simulink model "Tactor_NoTask _bkp"  (R2022b)
settings: Solver=FixedStepDiscrete  StartTime=0.0  StopTime=Inf  FixedStep=0.001  RelTol=1e-3  EnableMultiTasking=on
PreLoadFcn:
  | parambus = Simulink.Bus;
  | idx = 0;
  | 
  | idx = idx + 1;
  | parambus.Elements(idx) = Simulink.BusElement;
  | parambus.Elements(idx).Name = 'StimOn';
  | parambus.Elements(idx).DataType = 'uint8';
  | parambus.Elements(idx).Dimensions = [1, 1];
  | 
  | idx = idx + 1;
  | parambus.Elements(idx) = Simulink.BusElement;
  | parambus.Elements(idx).Name = 'DelayPeriod';
  | parambus.Elements(idx).DataType = 'uint16';
  | parambus.Elements(idx).Dimensions = [1, 2];
  | 
  | idx = idx + 1;
  | parambus.Elements(idx) = Simulink.BusElement;
  | parambus.Elements(idx).Name = 'StimDuration';
  | parambus.Elements(idx).DataType = 'uint16';
  | parambus.Elements(idx).Dimensions = [1, 1];
  | 
  | %%
  | 
  | FileLoggerEntry = Simulink.Bus;
  | FileLoggerEntry.Elements(1) = Simulink.BusElement;
  | FileLoggerEntry.Elements(1).Name = 'FileType';
  | FileLoggerEntry.Elements(1).DataType = 'uint8';
  | FileLoggerEntry.Elements(1).Dimensions = [1, 1];
  | FileLoggerEntry.Elements(2) = Simulink.BusElement;
  | FileLoggerEntry.Elements(2).Name = 'FieldName';
  | FileLoggerEntry.Elements(2).DataType = 'uint8';
  | FileLoggerEntry.Elements(2).Dimensions = [1, 20];
  | FileLoggerEntry.Elements(3) = Simulink.BusElement;
  | FileLoggerEntry.Elements(3).Name = 'DataType';
  | FileLoggerEntry.Elements(3).DataType = 'uint8';
  | FileLoggerEntry.Elements(3).Dimensions = [1, 6];
  | FileLoggerEntry.Elements(4) = Simulink.BusElement;
  | FileLoggerEntry.Elements(4).Name = 'NumElements';
  | FileLoggerEntry.Elements(4).DataType = 'uint8';
  | FileLoggerEntry.Elements(4).Dimensions = [1, 1];
  | FileLoggerEntry.Elements(5) = Simulink.BusElement;
  | FileLoggerEntry.Elements(5).Name = 'Data';
  | FileLoggerEntry.Elements(5).DataType = 'double';
  | FileLoggerEntry.Elements(5).Dimensions = [1, 255];
undefined symbols (not defined in the file): Ended, Single
libraries: slrealtimeiplib x6, speedgoatlib_IO191 x3, slrealtimeseriallib x2
settings Model: Creator=irwin  LastModifiedBy=l-zirwin
settings SolverCC: ConcurrentTasks=on  AlgebraicLoopSolver=TrustRegion  PositivePriorityOrder=on  InsertRTBMode=Never (minimum delay)
settings DataIOCC: SaveFormat=Array  SaveState=on  SignalLoggingName=logsOut
settings OptimizationCC: BlockReduction=off  BooleanDataType=off  OptimizeBlockIOStorage=off  BufferReuse=off  GlobalBufferReuse=off  ExpressionFolding=off  LocalBlockOutputs=off  InitFltsAndDblsToZero=on  OptimizeDataStoreBuffers=off  BusAssignmentInplaceUpdate=off
settings DebuggingCC: SaveWithParameterizedLinksMsg=none  UnderspecifiedInitializationDetection=Classic  MergeDetectMultiDrivingBlocksExec=none  CheckExecutionContextPreStartOutputMsg=on  SignalResolutionControl=TryResolveAllWithWarning  TasksWithSamePriorityMsg=none  UnconnectedInputMsg=warning  UnconnectedOutputMsg=warning  UnconnectedLineMsg=warning  SFUnexpectedBacktrackingDiag=warning  SFNoUnconditionalDefaultTransitionDiag=warning  SFExecutionAtInitializationDiag=none  SFMachineParentedDataDiag=warning  ArithmeticOperatorsInVariantConditions=warning
settings HardwareCC: ProdBitPerLong=64  ProdLongLongMode=on  ProdHWDeviceType=Intel->x86-64 (Linux 64)
settings ModelReferenceCC: EnableRefExpFcnMdlSchedulingChecks=on  PropagateSignalLabelsOutOfModel=off
settings SFSimCC: SimUseLocalCustomCode=off  SimTargetLang=C++
settings RTWCC: Description=Simulink Real-Time  SystemTargetFile=slrealtime.tlc  TemplateMakefile=slrealtime_default_tmf  RTWUseLocalCustomCode=off  Toolchain=Simulink Real-Time Toolchain  BuildConfiguration=Faster Runs  CodeExecutionProfiling=on  TargetLang=C++  DLArmComputeVersion=19.05
settings CodeAppCC: StateflowObjectComments=on
settings SimulinkRealTimeTargetCC: MATLABClassNameForMDSCustomization=Simulink.SoftwareTarget.GRTCustomization  UseGCCFastMath=on
settings ConfigComp: CovMetricSettings=dw  CovSaveCumulativeToWorkspaceVar=on  CovSaveSingleToWorkspaceVar=on  CovExternalEMLEnable=off  CovSFcnEnable=off

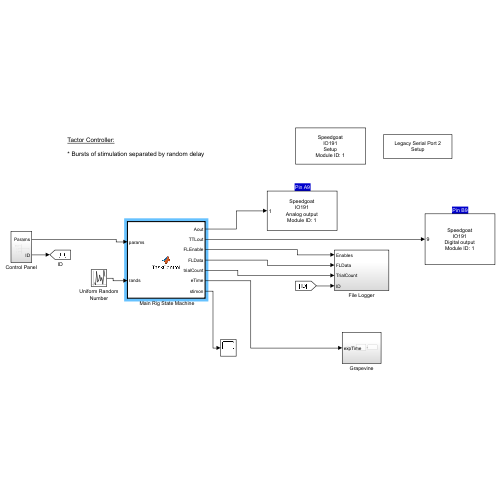
[thumbnail: Simulink's stored preview of the top-level diagram]
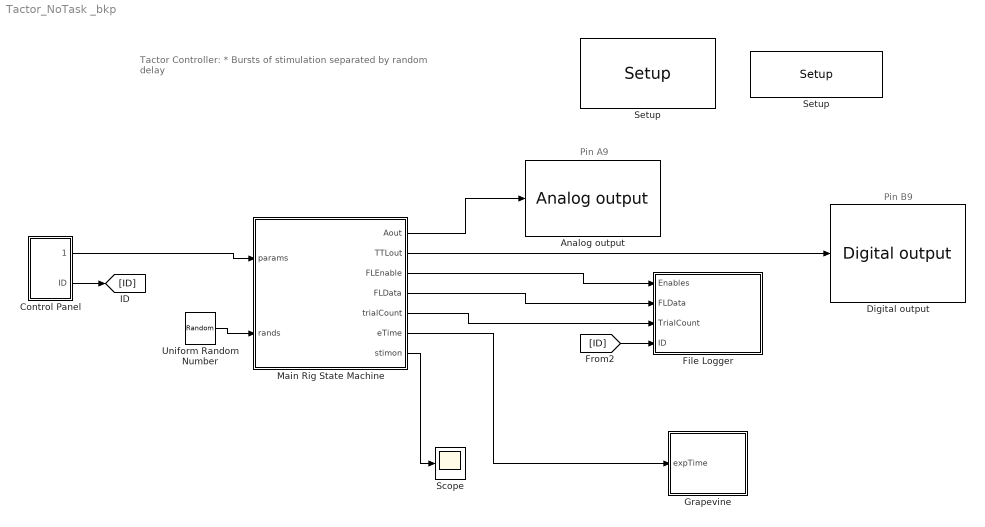
== system Tactor_NoTask _bkp ==
  note: Pin A9
  note: Pin B9
  note: Tactor Controller:
      |
      | * Bursts of stimulation separated by random delay
  " Main Rig State Machine" : MATLAB Function  TreatAsAtomicUnit=on
  "Analog output " : speedgoatlib_IO191/Analog output   parModuleId=1  parSampleTime=-1  parPciSlot=-1  parDacChannels=1  parModuleType=1  parDacRanges=5  parDacInitValues=0  parDacResets=1
      settings: SourceProductName=Simulink Real-Time: Speedgoat I/O Blockset
  Control Panel : Subsystem
  "Digital output " : speedgoatlib_IO191/Digital output   parModuleId=1  parSampleTime=-1  parPciSlot=-1  parDoChannels=9  parDoInitValues=0  parDoResets=1
      settings: SourceProductName=Simulink Real-Time: Speedgoat I/O Blockset
  File Logger : Subsystem
  Grapevine : Subsystem
  Scope : Scope
  Setup : slrealtimeseriallib/Mainboard/Setup  port=Legacy Serial Port 2  baud=115200  width=8  nstop=1  parity=None  ctsmode=off
  "Setup " : speedgoatlib_IO191/Setup   parModuleId=1  parPciSlot=-1  parTriggerSignal=TTL  parAdcChannels=1  parAdcRanges=3  parAdcChannel1=on  parAdcChannel2=off  parAdcChannel3=off  parAdcChannel4=off  parAdcChannel5=off  parAdcChannel6=off  parAdcChannel7=off  parAdcChannel8=off  parAdcMode=Single-Ended  parAdcRate=100000  parAdcRange11=+-10.24 V  parAdcRange21=+-24.576 V  parAdcRange12=+-10.24 V  parAdcRange22=+-24.576 V  parAdcRange13=+-10.24 V  parAdcRange23=+-24.576 V  parAdcRange14=+-10.24 V  parAdcRange24=+-24.576 V  parAdcRange15=+-10.24 V  parAdcRange25=+-24.576 V  parAdcRange16=+-10.24 V  parAdcRange26=+-24.576 V  parAdcRange17=+-10.24 V  parAdcRange27=+-24.576 V  parAdcRange18=+-10.24 V  parAdcRange28=+-24.576 V  parDacChannels=1  parDacChannel1=on  parDacChannel2=off  parDacChannel3=off  parDacChannel4=off  parDacMode=Single-Ended  parDacRanges=5  parDacInitValues=0  parDacResets=1  parDacRange1=+-2.5 V  parDacInitValue1=0  parDacReset1=on  parDacRange2=+-10 V  parDacInitValue2=0  parDacReset2=on  parDacRange3=+-10 V  parDacInitValue3=0  parDacReset3=on  parDacRange4=+-10 V  parDacInitValue4=0  parDacReset4=on  parDiChannels=[1 2 3 4 5 6 7 8 10 11 12 13 14 15 16]  parDoChannels=9  parDioFirstControl=2  parDioSecondControl=0  parDioChannel1=In  parExtra1=I  parExtra2=I  parExtra3=I  parDioChannel2=Out  parDioChannel3=In  parDioChannel4=In  parDioChannel5=In  parDioChannel6=In  parDioChannel7=In  parDioChannel8=In  parDioChannel9=In  parDoInitValues=[0 0 0 0]  parDoResets=[1 1 1 1]  parDoInitValue1=0  parDoReset1=on  parDoInitValue2=0  parDoReset2=on  parDoInitValue3=0  parDoReset3=on  parDoInitValue4=0  parDoReset4=on  parDoInitValue5=0  parDoReset5=on  parDoInitValue6=0  parDoReset6=on  parDoInitValue7=0  parDoReset7=on  parDoInitValue8=0  parDoReset8=on  parDoInitValue9=0  parDoReset9=on  parDoInitValue10=0  parDoReset10=on  parDoInitValue11=0  parDoReset11=on  parDoInitValue12=0  parDoReset12=on  parDoInitValue13=0  parDoReset13=on  parDoInitValue14=0  parDoReset14=on  parDoInitValue15=0  parDoReset15=on  parDoInitValue16=0  parDoReset16=on
      settings: SourceProductName=Simulink Real-Time: Speedgoat I/O Blockset
  Uniform Random Number : UniformRandomNumber  Minimum=[0]  Maximum=[1]  SampleTime=.001
  wires:
  " Main Rig State Machine"/3(FLEnable) -> File Logger/1(Enables)
  " Main Rig State Machine"/4(FLData) -> File Logger/2(FLData)
  " Main Rig State Machine"/5(trialCount) -> File Logger/3(TrialCount)
  Control Panel/2(ID) -> [ID]
  [ID] -> File Logger/4(ID)
  Control Panel/1(Params) -> " Main Rig State Machine"/1(params)
  Uniform Random Number/1 -> " Main Rig State Machine"/2(rands)
  " Main Rig State Machine"/1(Aout) -> "Analog output "/1
  " Main Rig State Machine"/2(TTLout) -> "Digital output "/1
  " Main Rig State Machine"/6(eTime) -> Grapevine/1(expTime)
  " Main Rig State Machine"/7(stimon) -> Scope/1

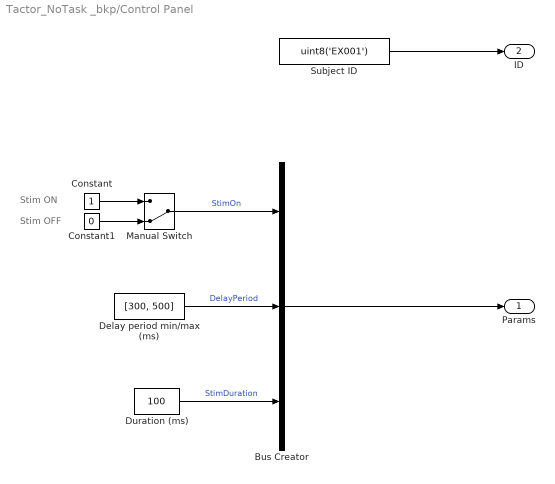
== system Tactor_NoTask _bkp/Control Panel ==
  note: Stim ON
  note: Stim OFF
  Bus Creator : BusCreator  Inputs=3  OutDataTypeStr=Bus: parambus  NonVirtualBus=on
  Constant : Constant  OutDataTypeStr=uint8
  Constant1 : Constant  Value=0  OutDataTypeStr=uint8
  Delay period min/max (ms) : Constant  Value=[300, 500]  OutDataTypeStr=uint16
  Duration (ms) : Constant  Value=100  OutDataTypeStr=uint16
  Manual Switch : ManualSwitch  CurrentSetting=0
  Subject ID : Constant  Value=uint8('EX001')  OutDataTypeStr=uint8
  Params : Outport
  ID : Outport  Port=2
  wires:
  Delay period min/max (ms)/1 -> Bus Creator/2  "DelayPeriod"
  Manual Switch/1 -> Bus Creator/1  "StimOn"
  Constant1/1 -> Manual Switch/2
  Constant/1 -> Manual Switch/1
  Bus Creator/1 -> Params/1
  Duration (ms)/1 -> Bus Creator/3  "StimDuration"
  Subject ID/1 -> ID/1

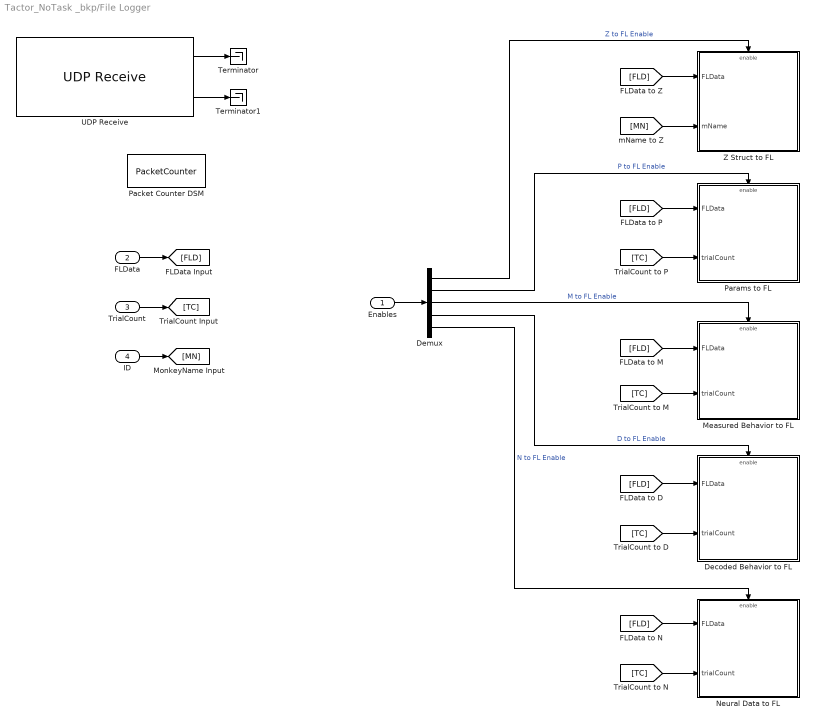
== system Tactor_NoTask _bkp/File Logger ==
  Enables : Inport  OutDataTypeStr=uint8  PortDimensions=[1 5]
  FLData : Inport  Port=2  OutDataTypeStr=Bus: FileLoggerEntry
  TrialCount : Inport  Port=3
  ID : Inport  Port=4
  Decoded Behavior to FL : Subsystem
  Demux : Demux  Outputs=5
  Measured Behavior to FL : Subsystem
  Neural Data to FL : Subsystem
  Packet Counter DSM : DataStoreMemory  DataStoreName=PacketCounter  WriteAfterWriteMsg=warning  ShowAdditionalParam=off  OutDataTypeStr=uint32  Dimensions=1
  Params to FL : Subsystem
  Terminator : Terminator
  Terminator1 : Terminator
  UDP Receive : slrealtimeiplib/UDP Receive  useHostTargetConn=off  ipAddress='192.168.8.1'  localPort=11114  rcvWidth=16  rcvFmAny=off  fmAddress='192.168.8.7'  sampleTime=-1  enableMessage=off  maxPackets=1
  Z Struct to FL : Subsystem
  wires:
  TrialCount/1 -> [TC]
  FLData/1 -> [FLD]
  [FLD] -> Z Struct to FL/1(FLData)
  [FLD] -> Params to FL/1(FLData)
  [FLD] -> Measured Behavior to FL/1(FLData)
  [FLD] -> Decoded Behavior to FL/1(FLData)
  [FLD] -> Neural Data to FL/1(FLData)
  [TC] -> Params to FL/2(trialCount)
  [TC] -> Measured Behavior to FL/2(trialCount)
  [TC] -> Decoded Behavior to FL/2(trialCount)
  [TC] -> Neural Data to FL/2(trialCount)
  Enables/1 -> Demux/1
  Demux/3 -> Measured Behavior to FL/Enable  "M to FL Enable"
  Demux/4 -> Decoded Behavior to FL/Enable  "D to FL Enable"
  Demux/5 -> Neural Data to FL/Enable  "N to FL Enable"
  Demux/2 -> Params to FL/Enable  "P to FL Enable"
  Demux/1 -> Z Struct to FL/Enable  "Z to FL Enable"
  ID/1 -> [MN]
  [MN] -> Z Struct to FL/2(mName)
  UDP Receive/2 -> Terminator1/1
  UDP Receive/1 -> Terminator/1

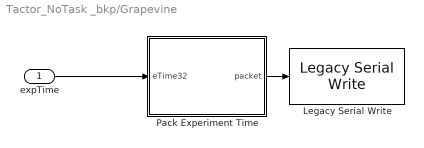
== system Tactor_NoTask _bkp/Grapevine ==
  expTime : Inport
  Legacy Serial Write : slrealtimeseriallib/Mainboard/Legacy Serial Write  port=Legacy Serial Port 2  dtype=count+32 bit uint  sampletime=-1
  Pack Experiment Time : MATLAB Function  TreatAsAtomicUnit=on
  wires:
  expTime/1 -> Pack Experiment Time/1(eTime32)
  Pack Experiment Time/1(packet) -> Legacy Serial Write/1

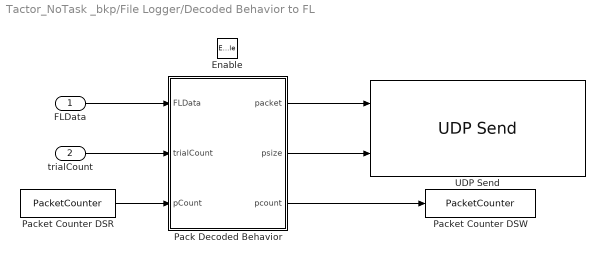
== system Tactor_NoTask _bkp/File Logger/Decoded Behavior to FL ==
  FLData : Inport
  trialCount : Inport  Port=2
  Enable : EnablePort
  Pack Decoded Behavior : MATLAB Function  TreatAsAtomicUnit=on
  Packet Counter DSR : DataStoreRead  DataStoreName=PacketCounter  SampleTime=.001  IndexOptions=Index vector (dialog)  Indices=1  OutputSizes=1
  Packet Counter DSW : DataStoreWrite  DataStoreName=PacketCounter  IndexOptions=Index vector (dialog)  Indices=1  OutputSizes=1
  UDP Send : slrealtimeiplib/UDP Send  useHostTargetConn=off  toAddress='192.168.8.7'  toPort=11114  sampleTime=-1  enableMessage=off  ipAddress='192.168.8.1'  localPort=11114
  wires:
  FLData/1 -> Pack Decoded Behavior/1(FLData)
  trialCount/1 -> Pack Decoded Behavior/2(trialCount)
  Packet Counter DSR/1 -> Pack Decoded Behavior/3(pCount)
  Pack Decoded Behavior/1(packet) -> UDP Send/1
  Pack Decoded Behavior/3(pcount) -> Packet Counter DSW/1
  Pack Decoded Behavior/2(psize) -> UDP Send/2

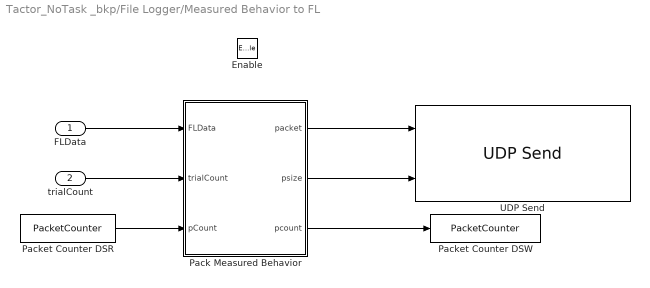
== system Tactor_NoTask _bkp/File Logger/Measured Behavior to FL ==
  FLData : Inport
  trialCount : Inport  Port=2
  Enable : EnablePort
  Pack Measured Behavior : MATLAB Function  TreatAsAtomicUnit=on
  Packet Counter DSR : DataStoreRead  DataStoreName=PacketCounter  SampleTime=.001  IndexOptions=Index vector (dialog)  Indices=1  OutputSizes=1
  Packet Counter DSW : DataStoreWrite  DataStoreName=PacketCounter  IndexOptions=Index vector (dialog)  Indices=1  OutputSizes=1
  UDP Send : slrealtimeiplib/UDP Send  useHostTargetConn=off  toAddress='192.168.8.7'  toPort=11114  sampleTime=-1  enableMessage=off  ipAddress='192.168.8.1'  localPort=11114
  wires:
  FLData/1 -> Pack Measured Behavior/1(FLData)
  trialCount/1 -> Pack Measured Behavior/2(trialCount)
  Packet Counter DSR/1 -> Pack Measured Behavior/3(pCount)
  Pack Measured Behavior/3(pcount) -> Packet Counter DSW/1
  Pack Measured Behavior/1(packet) -> UDP Send/1
  Pack Measured Behavior/2(psize) -> UDP Send/2

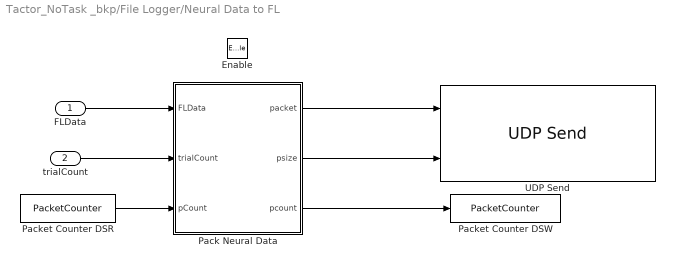
== system Tactor_NoTask _bkp/File Logger/Neural Data to FL ==
  FLData : Inport
  trialCount : Inport  Port=2
  Enable : EnablePort
  Pack Neural Data : MATLAB Function  TreatAsAtomicUnit=on
  Packet Counter DSR : DataStoreRead  DataStoreName=PacketCounter  SampleTime=.001  IndexOptions=Index vector (dialog)  Indices=1  OutputSizes=1
  Packet Counter DSW : DataStoreWrite  DataStoreName=PacketCounter  IndexOptions=Index vector (dialog)  Indices=1  OutputSizes=1
  UDP Send : slrealtimeiplib/UDP Send  useHostTargetConn=off  toAddress='192.168.8.7'  toPort=11114  sampleTime=-1  enableMessage=off  ipAddress='192.168.8.1'  localPort=11114
  wires:
  FLData/1 -> Pack Neural Data/1(FLData)
  trialCount/1 -> Pack Neural Data/2(trialCount)
  Packet Counter DSR/1 -> Pack Neural Data/3(pCount)
  Pack Neural Data/3(pcount) -> Packet Counter DSW/1
  Pack Neural Data/1(packet) -> UDP Send/1
  Pack Neural Data/2(psize) -> UDP Send/2

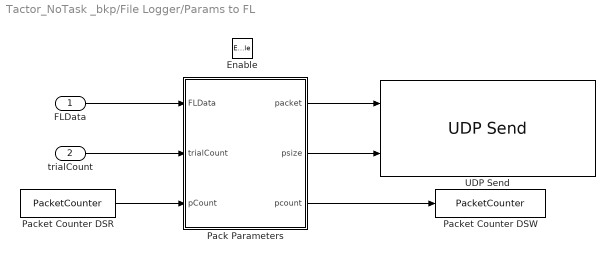
== system Tactor_NoTask _bkp/File Logger/Params to FL ==
  FLData : Inport
  trialCount : Inport  Port=2
  Enable : EnablePort
  Pack Parameters : MATLAB Function  TreatAsAtomicUnit=on
  Packet Counter DSR : DataStoreRead  DataStoreName=PacketCounter  SampleTime=.001  IndexOptions=Index vector (dialog)  Indices=1  OutputSizes=1
  Packet Counter DSW : DataStoreWrite  DataStoreName=PacketCounter  IndexOptions=Index vector (dialog)  Indices=1  OutputSizes=1
  UDP Send : slrealtimeiplib/UDP Send  useHostTargetConn=off  toAddress='192.168.8.7'  toPort=11114  sampleTime=-1  enableMessage=off  ipAddress='192.168.8.1'  localPort=11114
  wires:
  FLData/1 -> Pack Parameters/1(FLData)
  trialCount/1 -> Pack Parameters/2(trialCount)
  Packet Counter DSR/1 -> Pack Parameters/3(pCount)
  Pack Parameters/1(packet) -> UDP Send/1
  Pack Parameters/2(psize) -> UDP Send/2
  Pack Parameters/3(pcount) -> Packet Counter DSW/1

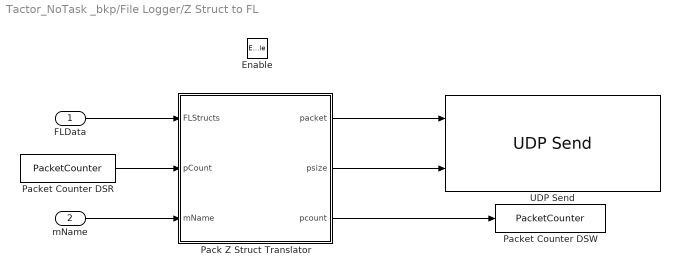
== system Tactor_NoTask _bkp/File Logger/Z Struct to FL ==
  FLData : Inport
  mName : Inport  Port=2
  Enable : EnablePort
  Pack Z Struct Translator : MATLAB Function  TreatAsAtomicUnit=on
  Packet Counter DSR : DataStoreRead  DataStoreName=PacketCounter  SampleTime=.001  IndexOptions=Index vector (dialog)  Indices=1  OutputSizes=1
  Packet Counter DSW : DataStoreWrite  DataStoreName=PacketCounter  IndexOptions=Index vector (dialog)  Indices=1  OutputSizes=1
  UDP Send : slrealtimeiplib/UDP Send  useHostTargetConn=off  toAddress='192.168.8.7'  toPort=11114  sampleTime=-1  enableMessage=off  ipAddress='192.168.8.1'  localPort=11114
  wires:
  FLData/1 -> Pack Z Struct Translator/1(FLStructs)
  Packet Counter DSR/1 -> Pack Z Struct Translator/2(pCount)
  mName/1 -> Pack Z Struct Translator/3(mName)
  Pack Z Struct Translator/3(pcount) -> Packet Counter DSW/1
  Pack Z Struct Translator/1(packet) -> UDP Send/1
  Pack Z Struct Translator/2(psize) -> UDP Send/2

== matlab function Tactor_NoTask _bkp/Grapevine/Pack Experiment Time ==
  data: eTime32 input uint32 size=1; packet output uint32 size=[1,5]
function packet = TypecastETime(eTime32)


packet = uint32([4, typecast(eTime32, 'uint8')]);

== matlab function Tactor_NoTask _bkp/ Main Rig State Machine ==
  data: Aout output double size=1; TTLout output double size=1; params input; rands input; FLEnable output; FLData output Bus: FileLoggerEntry; trialCount output; eTime output uint32 size=1; stimon output
function [Aout, TTLout, FLEnable, FLData, trialCount, eTime, stimon] = TaskControl(params, rands)

persistent exp_state trial_state exp_time trial_time trial_count intparams extparams...
           FLStruct

if (isempty(exp_state))
    exp_state = uint8(0);           % Experiment state variable
    trial_state = uint8(0);         % Trial state variable
    exp_time = uint32(0);           % Current experiment time
    trial_time = uint32(0);         % Current trial time
    trial_count = uint16(0);        % Count of the trials in the current run
    extparams = params;             % Initialize parameters to incoming struct
    FLStruct = genFLStruct();       % Struct array for File Logger data

    intparams = struct('DelayTime', uint16(0), ...          % delay period (ms)
                       'BlankTrial', uint8(0));          % indicator that stim was turned off

end

%%%%%%%%%%%%%%%%%%%%%%%%%%%%%%% Defines %%%%%%%%%%%%%%%%%%%%%%%%%%%%%%%%%%%

% Experiment states:
estate = struct('INIT', uint8(0), ...
                'RUN', uint8(1));

% Trial states:
tstate = struct('INIT',  uint8(0), ...
                'STIM',  uint8(1), ...
                'DELAY', uint8(2), ...
                'BLANK', uint8(3), ...
                'END',   uint8(4));

% File Logger TX enables:
fenable = struct('ZENABLE', uint8(1), ...
                 'TENABLE', uint8(2), ...
                 'MENABLE', uint8(3), ...
                 'DENABLE', uint8(4), ...
                 'NENABLE', uint8(5));

%%%%%%%%%%%%%%%%%%%%%%%%% Per-timestep updates %%%%%%%%%%%%%%%%%%%%%%%%%%%%

exp_time = exp_time + uint32(1);     % Update simulation time (1 ms per function call)
trial_time = trial_time + 1; % Update trial time

FLEnable = zeros(1,5,'uint8'); % Initialize file logger enables for this timestep

Aout = 0;
TTLout = 0;

%%%%%%%%%%%%%%%%%%%%%%% Stateflow switch statement %%%%%%%%%%%%%%%%%%%%%%%%

switch exp_state % Primary taskflow (experiment)
    case estate.INIT      % Initializing the File Logger
        
        %Send Z struct translator to File Logger:
        FLEnable(fenable.ZENABLE) = uint8(1);
        
        trial_state = tstate.INIT;
        exp_state = estate.RUN;

    case estate.RUN      % Run the experiment
        switch trial_state % Secondary taskflow (per trial)

            case tstate.INIT

                %Pick up changes to trial parameters:
                extparams = params;
                
                % Determine delay period time:
                intparams.DelayTime = uint16(rands(1)*double(diff(extparams.DelayPeriod)) + double(extparams.DelayPeriod(1)));

                % Blank recording trial while stim is turned off:
                intparams.BlankTrial = uint8(~extparams.StimOn);
                
                % Update File Logger struct with new trial params:
                FLStruct = updateFLParams(FLStruct, extparams, intparams);
                
                % Send trial parameters to File Logger:
                FLEnable(fenable.TENABLE) = uint8(1);
                
                if (intparams.BlankTrial)
                    trial_state = tstate.BLANK;
                else
                    trial_state = tstate.STIM;
                end

                trial_count = trial_count + uint16(1);
                trial_time = uint32(0);

            case tstate.STIM

                % Generate ongoing sine wave based on trial time:
                TTLout = 1;
                Aout = 0.167 * sin(2*pi*100*double(trial_time)/1000);

                % Test for complete stim period:
                if (trial_time >= extparams.StimDuration)
                    trial_state = tstate.DELAY;
                end
                
                % End the trial if experimenter turns off stim:
                if (~params.StimOn)
                    trial_state = tstate.END;
                end

                %Update behavior/neural File Logger structs:
                FLStruct = updateFLData(FLStruct, [], [], [], exp_time);
                
                %Send measured behavior to File Logger:
                FLEnable([fenable.MENABLE]) = uint8(1);

            case tstate.DELAY

                % Output zero

                % Test for complete delay period:
                if (trial_time >= extparams.StimDuration + intparams.DelayTime)
                    trial_state = tstate.END;
                end

                % End the trial if experimenter turns off stim:
                if (~params.StimOn)
                    trial_state = tstate.END;
                end

                %Update behavior/neural File Logger structs:
                FLStruct = updateFLData(FLStruct, [], [], [], exp_time);
                
                %Send measured behavior + Neural to File Logger:
                FLEnable([fenable.MENABLE]) = uint8(1);
            
            case tstate.BLANK

                % Test for complete stim and delay period:
                if (trial_time >= extparams.StimDuration + intparams.DelayTime)
                    trial_state = tstate.END;
                end
                
                % End the trial is experimenter turns stim on again:
                if (params.StimOn)
                    trial_state = tstate.END;
                end

                %Update behavior/neural File Logger structs:
                FLStruct = updateFLData(FLStruct, [], [], [], exp_time);
                
                %Send measured behavior + Neural to File Logger:
                FLEnable([fenable.MENABLE]) = uint8(1);

            case tstate.END

                % Update File Logger struct with trial wrap-up data:
                FLStruct = updateFLParams(FLStruct, extparams, intparams);

                % Send trial parameters to File Logger:
                FLEnable(fenable.TENABLE) = uint8(1);

                % Start a new trial:
                trial_state = tstate.INIT;
        end
end


%%%%%%%%%%%%%%%%%%%%%%%% Assign Output Variables: %%%%%%%%%%%%%%%%%%%%%%%%%

FLData = FLStruct;

trialCount = trial_count;
eTime = exp_time;
stimon = extparams.StimOn;
end

%%%%%%%%%%%%%%%%%%%%%%%%%%% Helper Functions: %%%%%%%%%%%%%%%%%%%%%%%%%%%%%

% Initializes an array of structures for output to the File Logger:
function flStructs = genFLStruct()

%Set up initial structure for a FileLoggerEntry struct:
tempStructs = struct('FileType', uint8(0), 'FieldName', uint8(zeros(1,20)), ...
    'DataType', uint8(zeros(1,6)), 'NumElements', uint8(0), 'Data', zeros(1,255));

%Replicate N times (#params + #behavior [meas/dec] + #neural):
flStructs = repmat(tempStructs, 1, 10);

%File types:
ftype = struct('BEHAVIOR_MEAS', uint8(2), ...
               'BEHAVIOR_DEC', uint8(3), ...
               'DATA_NEUR', uint8(4), ...
               'PARAM_START', uint8(5), ...
               'PARAM_END', uint8(6));

%Set fieldnames, file types, data types:
flStructs(1) = getStruct(ftype.PARAM_START, 'DelayTime', 'uint16', 1, []);
flStructs(2) = getStruct(ftype.PARAM_START, 'StimDuration', 'uint16', 1, []);
flStructs(3) = getStruct(ftype.PARAM_START, 'BlankTrial', 'uint8', 1, []);
flStructs(4) = getStruct(ftype.BEHAVIOR_MEAS, 'ExperimentTime', 'single', 1, []);

end


% Updates the File Logger array with new parameters:
function flStructs = updateFLParams(flStruct_old, extparams, intparams)

%extparams = External, tunable parameters; intparams = Internal parameters.
%e.g. extparam1 = User-set TargetScaling, intparam1 = program-set TargetLoc.

flStructs = flStruct_old;
flStructs(1).Data(1:length(intparams.DelayTime))      = double(intparams.DelayTime);
flStructs(2).Data(1:length(extparams.StimDuration))   = double(extparams.StimDuration);
flStructs(3).Data(1:length(intparams.BlankTrial))     = double(intparams.BlankTrial);

end

% Updates the File Logger array with new behavior/neural data:
function flStructs = updateFLData(flStruct_old, mBehavior, dBehavior, neural, eTime)

flStructs = flStruct_old;
flStructs(4).Data(1:length(eTime))     = double(eTime);

end

% Helper function to create an FL struct from inputs:
function ret = getStruct(filetype,fieldname,datatype,numel,data)

ft = uint8(filetype);                                   % FileType
fn = uint8([fieldname, zeros(1,20-length(fieldname))]); % FieldName
dt = uint8([datatype, zeros(1,6-length(datatype))]);    % DataType
ne = uint8(numel);                                      % NumElements
d = double([data, zeros(1,255-length(data))]);          % Data

%Create and return structure:
ret = struct('FileType', ft, 'FieldName', fn, 'DataType', dt, 'NumElements', ne, 'Data', d);

end

== matlab function Tactor_NoTask _bkp/File Logger/Z Struct to FL/Pack Z Struct Translator ==
  data: packet output uint8 size=[1,1500]; FLStructs input Bus: FileLoggerEntry; pCount input uint32 size=1; psize output double size=1; mName input uint8; pcount output uint32 size=1
% This translates the FileLoggerEntry struct array to a Z struct description
% string for the Z Struct Translator script to use at a later date.
%
% FL Packet:[packetCount(4b), packetType(1b), data(xb)]
%   -> First 2 bytes of non-ZPacket data are the trialCount
%
% Z Struct descriptor: 'fieldname1-datatype1-numElements1-fieldname2-...'
%
%   Written by Zach Irwin for the Chestek Lab, 2012
%%%%%%%%%%%%%%%%%%%%%%%%%%%%%%%%%%%%%%%%%%%%%%%%%%%%%%%%%%%%%%%%%%%%%%%%%%%

function [packet, psize, pcount] = genZPacket(FLStructs, pCount, mName)
%#codegen

sb = uint8('-'); % Spacer byte
headers = uint8([':P:'; ':M:'; ':D:'; ':N:']); % File Type headers

%Current packet size (with headers/monkey name, max size = 1500 bytes):
psize = double(4 + 1 + length(mName) + 1);

%Initialize packet (packetCount, packetType, mNameSize, mName, padding):
packet = uint8([typecast(uint32(pCount), 'uint8'), uint8(0), uint8(length(mName)), mName',zeros(1,1500-psize)]);

%Sort FLStructs into FileTypes (Params, mBehavior, dBehavior, Neural):
idxs = zeros(5,length(FLStructs));

for i = 1:length(FLStructs)

     switch FLStructs(i).FileType
         case 2 % Measured Behavior File Type
             idxs(2, nnz(idxs(2,:)) + 1) = i;
         case 3 % Decoded Behavior File Type
             idxs(3, nnz(idxs(3,:)) + 1) = i;
         case 4 % Neural Data File Type
             idxs(4, nnz(idxs(4,:)) + 1) = i;
         case 5 % Trial Begin Parameter File Type
             idxs(1, nnz(idxs(1,:)) + 1) = i;
         case 6 % Trial End Parameter File Type
             idxs(5, nnz(idxs(1,:)) + 1) = i;
     end
    
end

%Iterate through each File Type, add data to packet:
for i = 1:4
    
    % Collect structs for the current File Type:
    nidxs = idxs(i, :); % Current set of indices for ith File Type
    
    if (i == 1)
        nidxs5 = idxs(5,:); % Indices for the End Parameters File Type
        data = [FLStructs(nidxs(nidxs~=0)), FLStructs(nidxs5(nidxs5~=0))];
    else
        data = FLStructs(nidxs(nidxs ~= 0)); % Current File Type Structs
    end
    
    % Add correct File Type header:
    start = psize + uint16(1); stop = psize + uint16(3);
    packet(start:stop) = headers(i,:);
    
    % Update number of elements in the packet:
    psize = psize + double(3);
    
    % Iterate through the File Type structs & add to packet:
    for j = 1:length(data)
        
        % Recover non-NULL fieldName string:
        fname = data(j).FieldName(data(j).FieldName ~= 0);
        
        % Recover non-NULL dataType string:
        dtype = data(j).DataType(data(j).DataType ~= 0);
        
        % If either of these is empty, generate an error:
        if (isempty(fname) || isempty(dtype))
            error('An FLStruct FieldName or DataType is NULL. Don''t include extraneous FLStructs.');
        end
        
        % Recover numElements byte:
        numel = data(j).NumElements;
        
        % Size of all of these elements + 3 spacer bytes:
        inum = length(fname) + length(dtype) + length(numel) + 3;
        
        % Pack this set of bytes into the packet:
        start = psize + uint16(1); stop = psize + uint16(inum);
        packet(start:stop) = uint8([fname, sb, dtype, sb, numel, sb]);
        
        % Update number of elements in the packet:
        psize = psize + double(inum);
        
    end
    
end

% Update packet count:
pcount = pCount + uint32(1);

end

== matlab function Tactor_NoTask _bkp/File Logger/Params to FL/Pack Parameters ==
  data: FLData input Bus: FileLoggerEntry; packet output uint8 size=[1,1500]; trialCount input uint16 size=1; pCount input uint32 size=1; psize output size=1; pcount output uint32 size=1
% This packs a vector of the trial parameters to send to the File Logger
%
% FL Packet:[runTime(4b), packetType(1b), data(xb)]
%   -> First 2 bytes of non-ZPacket data are the trialCount
%
%   Written by Zach Irwin for the Chestek Lab, 2012
%%%%%%%%%%%%%%%%%%%%%%%%%%%%%%%%%%%%%%%%%%%%%%%%%%%%%%%%%%%%%%%%%%%%%%%%%%%

function [packet, psize, pcount] = genPPacket(FLData, trialCount, pCount)
%#codegen

persistent prev_count

%This function gets called twice per trial, prev_count lets us know which
%type of trial parameters to send (FileType 5 or FileType 6)
if (isempty(prev_count))
    prev_count = -1;        
end

%Figure out which FileType to send:
if (prev_count == trialCount)
    ftype = 6;  %Send the Trial Wrap-up parameters
else
    ftype = 5;  %Send Trial Begin parameters
    prev_count = double(trialCount); %Reset count
end

%Convert runTime & trialCount to uint8 vectors:
rt = typecast(uint32(pCount), 'uint8');
tc = typecast(uint16(trialCount), 'uint8');

%Initialize packet vector [runTime(x4), packetType(x1), trialCount(x2), data(x1493)]:
packet = uint8([rt, uint8(ftype), tc, zeros(1,1493)]);

%Keep track of no. of bytes in the packet:
psize = double(7); %4 runTime bytes, 1 packetType byte, and 2 trialCount bytes

for i = 1:length(FLData)
    
    %Skip FLData structs without parameter data (fileType = 5 or 6):
   if (FLData(i).FileType ~= ftype)
       continue;
   end
   
   %Get non-zero data from struct:
   ddata = FLData(i).Data(1:FLData(i).NumElements); %Elements as doubles
   
   %Cast data to correct type, then uint8s for packing:
   type = char(FLData(i).DataType(FLData(i).DataType ~= 0));
   if (strcmp(type, 'uint8'))
       data = uint8(ddata);
   elseif (strcmp(type, 'int8'))
       data = typecast(int8(ddata),'uint8');
   elseif (strcmp(type, 'uint16'))
       data = typecast(uint16(ddata),'uint8');
   elseif (strcmp(type, 'int16'))
       data = typecast(int16(ddata),'uint8');
   elseif (strcmp(type, 'uint32'))
       data = typecast(uint32(ddata),'uint8');
   elseif (strcmp(type, 'int32'))
       data = typecast(int32(ddata),'uint8');
   elseif (strcmp(type, 'single'))
       data = typecast(single(ddata),'uint8');
   elseif (strcmp(type, 'double'))
       data = typecast(ddata,'uint8');
   else
       data = uint8(0); % Should never happen
   end
   
   %Add data to packet:
   start = psize + uint16(1); stop = psize + uint16(length(data));
   packet(start:stop) = data;
   
   %Update number of elements in the packet:
   psize = psize + double(length(data));
   
   if (psize > 1500)
       error('Packet size reached: P Packet type');
   end
   
end

%Update packet count:
pcount = pCount + uint32(1);
end

== matlab function Tactor_NoTask _bkp/File Logger/Measured Behavior to FL/Pack Measured Behavior ==
  data: FLData input Bus: FileLoggerEntry; packet output uint8 size=[1,1500]; trialCount input uint16 size=1; pCount input uint32 size=1; psize output size=1; pcount output uint32 size=1
% This packs a vector of the measured behavior to send to the File Logger
%
% FL Packet:[runTime(4b), packetType(1b), data(xb)]
%   -> First 2 bytes of non-ZPacket data are the trialCount
%
%   Written by Zach Irwin for the Chestek Lab, 2012
%%%%%%%%%%%%%%%%%%%%%%%%%%%%%%%%%%%%%%%%%%%%%%%%%%%%%%%%%%%%%%%%%%%%%%%%%%%

function [packet, psize, pcount] = genMPacket(FLData, trialCount, pCount)
%#codegen

%Convert runTime & trialCount to uint8 vectors:
rt = typecast(uint32(pCount), 'uint8');
tc = typecast(uint16(trialCount), 'uint8');

%Initialize packet vector [runTime(x4), packetType(x1), trialCount(x2), data(x1493)]:
packet = uint8([rt, uint8(2), tc, zeros(1,1493)]);

%Keep track of no. of bytes in the packet:
psize = double(7); %4 runTime bytes, 1 packetType byte, and 2 trialCount bytes

for i = 1:length(FLData)
    
    %Skip FLData strucuts without meas. behavior data (fileType = 2):
   if (FLData(i).FileType ~= 2)
       continue;
   end
   
   %Get non-zero data from struct:
   ddata = FLData(i).Data(1:FLData(i).NumElements); %Elements as doubles
   
   %Cast data to correct type, then uint8s for packing:
   type = char(FLData(i).DataType(FLData(i).DataType ~= 0));
   if (strcmp(type, 'uint8'))
       data = uint8(ddata);
   elseif (strcmp(type, 'int8'))
       data = typecast(int8(ddata),'uint8');
   elseif (strcmp(type, 'uint16'))
       data = typecast(uint16(ddata),'uint8');
   elseif (strcmp(type, 'int16'))
       data = typecast(int16(ddata),'uint8');
   elseif (strcmp(type, 'uint32'))
       data = typecast(uint32(ddata),'uint8');
   elseif (strcmp(type, 'int32'))
       data = typecast(int32(ddata),'uint8');
   elseif (strcmp(type, 'single'))
       data = typecast(single(ddata),'uint8');
   elseif (strcmp(type, 'double'))
       data = typecast(ddata,'uint8');
   else
       data = uint8(0); % Should never happen
   end
   
   %Add data to packet:
   start = psize + uint16(1); stop = psize + uint16(length(data));
   packet(start:stop) = data;
   
   %Update number of elements in the packet:
   psize = psize + double(length(data));
   
   if (psize > 1500)
       error('Packet size reached: M Packet type');
   end
   
end

%Update packet count:
pcount = pCount + uint32(1);
end

== matlab function Tactor_NoTask _bkp/File Logger/Decoded Behavior to FL/Pack Decoded Behavior ==
  data: FLData input Bus: FileLoggerEntry; packet output uint8 size=[1,1500]; trialCount input uint16 size=1; pCount input uint32 size=1; psize output size=1; pcount output uint32 size=1
% This packs a vector of the decoded behavior to send to the File Logger
%
% FL Packet:[runTime(4b), packetType(1b), data(xb)]
%   -> First 2 bytes of non-ZPacket data are the trialCount
%
%   Written by Zach Irwin for the Chestek Lab, 2012
%%%%%%%%%%%%%%%%%%%%%%%%%%%%%%%%%%%%%%%%%%%%%%%%%%%%%%%%%%%%%%%%%%%%%%%%%%%

function [packet, psize, pcount] = genDPacket(FLData, trialCount, pCount)
%#codegen

%Convert runTime & trialCount to uint8 vectors:
rt = typecast(uint32(pCount), 'uint8');
tc = typecast(uint16(trialCount), 'uint8');

%Initialize packet vector [runTime(x4), packetType(x1), trialCount(x2), data(x1493)]:
packet = uint8([rt, uint8(3), tc, zeros(1,1493)]);

%Keep track of no. of bytes in the packet:
psize = double(7); %4 runTime bytes, 1 packetType byte, and 2 trialCount bytes

for i = 1:length(FLData)
    
    %Skip FLData strucuts without dec. behavior data (fileType = 3):
   if (FLData(i).FileType ~= 3)
       continue;
   end
   
   %Get non-zero data from struct:
   ddata = FLData(i).Data(1:FLData(i).NumElements); %Elements as doubles
   
   %Cast data to correct type, then uint8s for packing:
   type = char(FLData(i).DataType(FLData(i).DataType ~= 0));
   if (strcmp(type, 'uint8'))
       data = uint8(ddata);
   elseif (strcmp(type, 'int8'))
       data = typecast(int8(ddata),'uint8');
   elseif (strcmp(type, 'uint16'))
       data = typecast(uint16(ddata),'uint8');
   elseif (strcmp(type, 'int16'))
       data = typecast(int16(ddata),'uint8');
   elseif (strcmp(type, 'uint32'))
       data = typecast(uint32(ddata),'uint8');
   elseif (strcmp(type, 'int32'))
       data = typecast(int32(ddata),'uint8');
   elseif (strcmp(type, 'single'))
       data = typecast(single(ddata),'uint8');
   elseif (strcmp(type, 'double'))
       data = typecast(ddata,'uint8');
   else
       data = uint8(0); % Should never happen
   end
   
   %Add data to packet:
   start = psize + uint16(1); stop = psize + uint16(length(data));
   packet(start:stop) = data;
   
   %Update number of elements in the packet:
   psize = psize + double(length(data));
   
   if (psize > 1500)
       error('Packet size reached: D Packet type');
   end
   
end

%Update packet count:
pcount = pCount + uint32(1);
end

== matlab function Tactor_NoTask _bkp/File Logger/Neural Data to FL/Pack Neural Data ==
  data: FLData input Bus: FileLoggerEntry; packet output uint8 size=[1,1500]; trialCount input uint16 size=1; pCount input uint32 size=1; psize output size=1; pcount output uint32 size=1
    % This packs a vector of the Neural data to send to the File Logger
%
% FL Packet:[runTime(4b), packetType(1b), data(xb)]
%   -> First 2 bytes of non-ZPacket data are the trialCount
%
% *NOTE: Neural packets have an "end packet" character(255) as the last
% byte in the packet. This is to support variable length spike channels.
%
%   Written by Zach Irwin for the Chestek Lab, 2012
%%%%%%%%%%%%%%%%%%%%%%%%%%%%%%%%%%%%%%%%%%%%%%%%%%%%%%%%%%%%%%%%%%%%%%%%%%%

function [packet, psize, pcount] = genNPacket(FLData, trialCount, pCount)
%#codegen

%Convert runTime & trialCount to uint8 vectors:
rt = typecast(uint32(pCount), 'uint8');
tc = typecast(uint16(trialCount), 'uint8');

%Initialize packet vector [runTime(x4), packetType(x1), trialCount(x2), data(x1493)]:
packet = uint8([rt, uint8(4), tc, zeros(1,1493)]);

%Keep track of no. of bytes in the packet:
psize = double(7); %4 runTime bytes, 1 packetType byte, and 2 trialCount bytes

for i = 1:length(FLData)
    
    %Skip FLData structs without neural data (fileType = 4):
   if (FLData(i).FileType ~= 4)
       continue;
   end
   
   %Get non-zero data from struct:
   if (FLData(i).NumElements == 0)
        ddata = FLData(i).Data(FLData(i).Data ~= 0); %Elements as doubles
   else
        ddata = FLData(i).Data(1:FLData(i).NumElements); %Elements as doubles
   end
   
   %Cast data to correct type, then uint8s for packing:
   type = char(FLData(i).DataType(FLData(i).DataType ~= 0));
   if (strcmp(type, 'uint8'))
       data = uint8(ddata);
   elseif (strcmp(type, 'int8'))
       data = typecast(int8(ddata),'uint8');
   elseif (strcmp(type, 'uint16'))
       data = typecast(uint16(ddata),'uint8');
   elseif (strcmp(type, 'int16'))
       data = typecast(int16(ddata),'uint8');
   elseif (strcmp(type, 'uint32'))
       data = typecast(uint32(ddata),'uint8');
   elseif (strcmp(type, 'int32'))
       data = typecast(int32(ddata),'uint8');
   elseif (strcmp(type, 'single'))
       data = typecast(single(ddata),'uint8');
   elseif (strcmp(type, 'double'))
       data = typecast(ddata,'uint8');
   else
       data = uint8(0); % Should never happen
   end
   
   %Add data to packet:
   start = psize + uint16(1); stop = psize + uint16(length(data));
   packet(start:stop) = data;
   
   %Update number of elements in the packet:
   psize = psize + double(length(data));
   
   if (psize >= 1500)
       error('Packet size reached: N Packet type');
   end
   
end

%Add End Packet byte:
packet(psize+uint16(1)) = uint8(255);
psize = psize + double(1);

%Update packet count:
pcount = pCount + uint32(1);

end
